simulink model "chap11_4sim"  (Simulink 7.0)
settings: Solver=ode45  StartTime=0.0  StopTime=30  RelTol=1e-3
settings Model: Creator=eleliuj  LastModifiedBy=eleliuj
settings DataIOCC: SignalLoggingName=sigsOut
settings DebuggingCC: SaveWithParameterizedLinksMsg=none  SignalResolutionControl=TryResolveAllWithWarning  SolverPrmCheckMsg=none  MultiTaskDSMMsg=warning  MultiTaskCondExecSysMsg=none  StrictBusMsg=None
settings HardwareCC: TargetUnknown=on
settings RTWCC: IncludeERTFirstTime=on

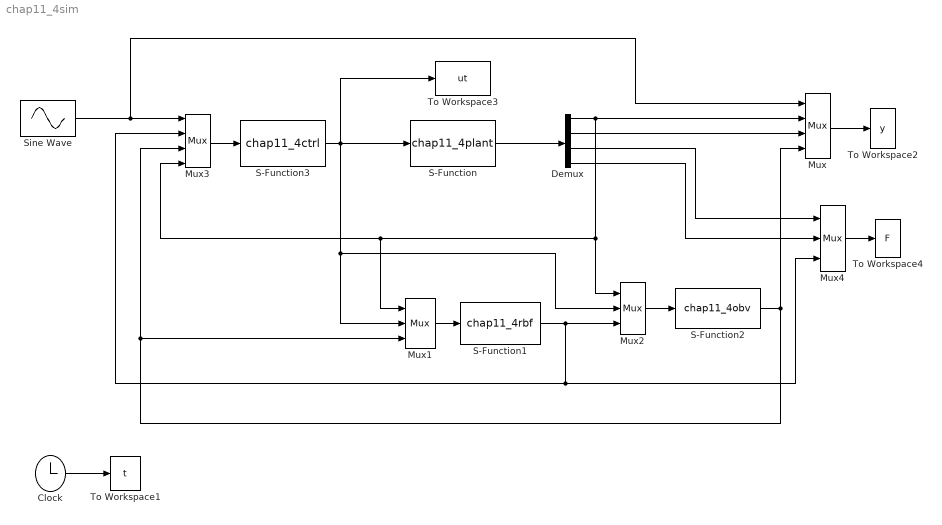
== system chap11_4sim ==
  Clock : Clock
      settings: Decimation=10
  Demux : Demux
  Mux : Mux
  Mux1 : Mux  Inputs=3
  Mux2 : Mux  Inputs=3
  Mux3 : Mux
  Mux4 : Mux  Inputs=3
  S-Function : S-Function  FunctionName=chap11_4plant
  S-Function1 : S-Function  FunctionName=chap11_4rbf
  S-Function2 : S-Function  FunctionName=chap11_4obv
  S-Function3 : S-Function  FunctionName=chap11_4ctrl
  Sine Wave : Sin  SampleTime=0
  To Workspace1 : ToWorkspace  VariableName=t  SampleTime=-1  SaveFormat=Array
  To Workspace2 : ToWorkspace  VariableName=y  SampleTime=-1  SaveFormat=Array
  To Workspace3 : ToWorkspace  VariableName=ut  SampleTime=-1  SaveFormat=Array
  To Workspace4 : ToWorkspace  VariableName=F  SampleTime=-1  SaveFormat=Array
  wires:
  Clock/1 -> To Workspace1/1
  Mux/1 -> To Workspace2/1
  S-Function2/1 -> Mux1/3, Mux3/3, Mux/4
  Mux1/1 -> S-Function1/1
  Mux2/1 -> S-Function2/1
  S-Function1/1 -> Mux2/3, Mux3/2, Mux4/3
  S-Function/1 -> Demux/1
  Demux/1 -> Mux2/1, Mux1/1, Mux3/4, Mux/2
  S-Function3/1 -> S-Function/1, Mux1/2, Mux2/2, To Workspace3/1
  Sine Wave/1 -> Mux3/1, Mux/1
  Mux3/1 -> S-Function3/1
  Demux/2 -> Mux/3
  Demux/3 -> Mux4/1
  Demux/4 -> Mux4/2
  Mux4/1 -> To Workspace4/1
